simulink model "chairforceoneMV"  (R2024a)
settings: Solver=VariableStepAuto  StartTime=0.0  StopTime=1000.0  RelTol=1e-3
settings Model: Creator=sprinkle  LastModifiedBy=suryachand
settings OptimizationCC: ReuseModelBlockBuffer=off
settings RTWCC: GPUComputeCapability=3.5

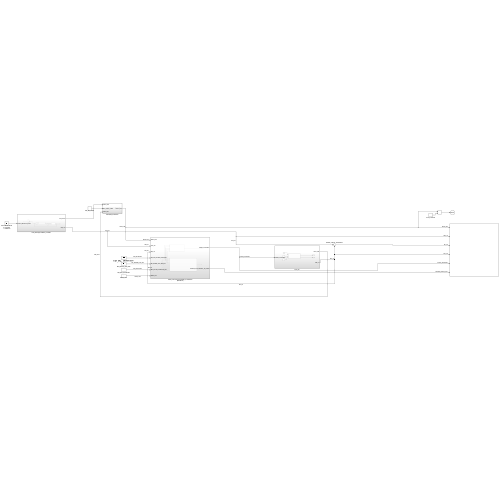
[thumbnail: Simulink's stored preview of the top-level diagram]
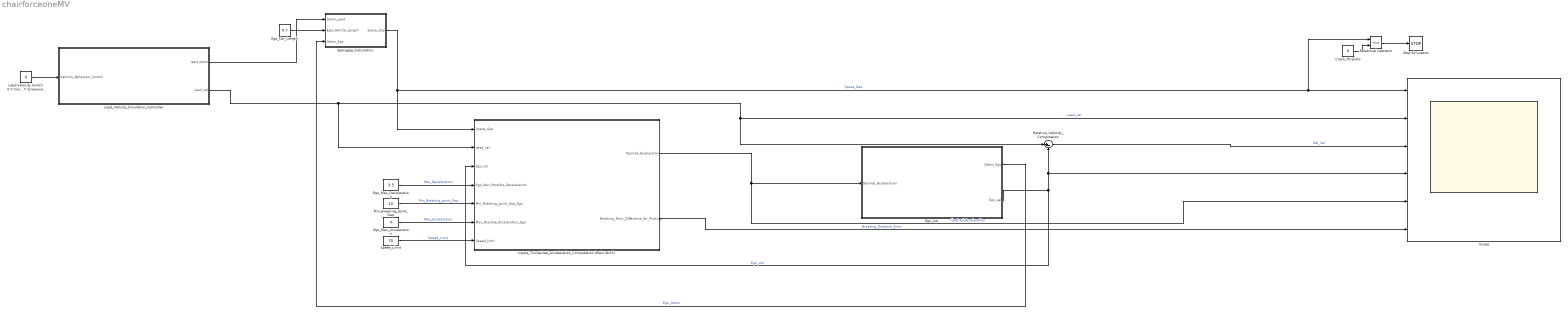
== system chairforceoneMV ==
  Crash_Thrshold : Constant  Value=0
  Ego_Car : Subsystem
  Ego_Car_Length : Constant  Value=4.7
  Ego_Max_Acceleration : Constant  Value=4
  "Ego_Max_Deceleration " : Constant  Value=3.5
  Inputs_To-Desired_Acceleration_Computation (Main Work) : Subsystem
  "Lead Velocity Switch 0 = Constant 1 = Sinewave " : Constant  Value=0
  Lead_Vehicle_Simulation_Controller : Subsystem
  Min_Breaking_point_Gap : Constant  Value=10
  Relational Operator : RelationalOperator  Operator=<=  OutDataTypeStr=boolean  RndMeth=Simplest  InputSameDT=off
  Relative_Velocity_Computation : Sum  Inputs=|+-
  Scope : Scope  NumInputPorts=6
  Spacegap_Calculation : Subsystem
  Speed_Limit : Constant  Value=70
  Stop Simulation : Stop
  wires:
  Relative_Velocity_Computation/1 -> Scope/3  "Rel_Vel"
  Lead_Vehicle_Simulation_Controller/2(lead_vel) -> Relative_Velocity_Computation/1, Scope/2, Inputs_To-Desired_Acceleration_Computation (Main Work)/2(Lead_vel)  "Lead_vel"
  "Lead Velocity Switch 0 = Constant 1 = Sinewave "/1 -> Lead_Vehicle_Simulation_Controller/1(Velocity_Behaviour_Switch)
  Spacegap_Calculation/1(Space_Gap) -> Inputs_To-Desired_Acceleration_Computation (Main Work)/1(Space_Gap), Relational Operator/1, Scope/1  "Space_Gap"
  Lead_Vehicle_Simulation_Controller/1(lead_odom) -> Spacegap_Calculation/1(Odom_Lead)
  Ego_Car_Length/1 -> Spacegap_Calculation/2(Ego_Vehicle_Length)
  Inputs_To-Desired_Acceleration_Computation (Main Work)/1(Desired_Acceleration) -> Scope/5, Ego_Car/1(Desired_Acceleration)  "Desired_Acceleration"
  "Ego_Max_Deceleration "/1 -> Inputs_To-Desired_Acceleration_Computation (Main Work)/4(Ego_Max_Possible_Deceleration)  "Max_Deceleration"
  Min_Breaking_point_Gap/1 -> Inputs_To-Desired_Acceleration_Computation (Main Work)/5(Min_Breaking_point_Gap_Ego)  "Min_Breaking_point_Gap"
  Ego_Car/2(Ego_vel) -> Relative_Velocity_Computation/2, Scope/4, Inputs_To-Desired_Acceleration_Computation (Main Work)/3(Ego_vel)  "Ego_Vel"
  Ego_Car/1(Odom_Ego) -> Spacegap_Calculation/3(Odom_Ego)  "Ego_Odom"
  Ego_Max_Acceleration/1 -> Inputs_To-Desired_Acceleration_Computation (Main Work)/6(Max_Possible_Acceleration_Ego)  "Max_Acceleration"
  Inputs_To-Desired_Acceleration_Computation (Main Work)/2(Breaking_Point_Difference_for_Plotting) -> Scope/6  "Breaking_Distance_Error"
  Speed_Limit/1 -> Inputs_To-Desired_Acceleration_Computation (Main Work)/7(Speed_limit)  "Speed_Limit"
  Relational Operator/1 -> Stop Simulation/1
  Crash_Thrshold/1 -> Relational Operator/2

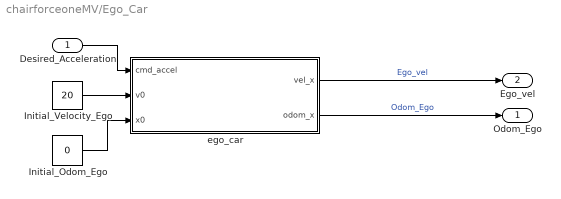
== system chairforceoneMV/Ego_Car ==
  Desired_Acceleration : Inport
  Initial_Odom_Ego : Constant  Value=0
  Initial_Velocity_Ego : Constant  Value=20
  ego_car : Subsystem
  Odom_Ego : Outport
  Ego_vel : Outport  Port=2
  wires:
  ego_car/2(odom_x) -> Odom_Ego/1  "Odom_Ego"
  ego_car/1(vel_x) -> Ego_vel/1  "Ego_vel"
  Initial_Odom_Ego/1 -> ego_car/3(x0)
  Desired_Acceleration/1 -> ego_car/1(cmd_accel)
  Initial_Velocity_Ego/1 -> ego_car/2(v0)

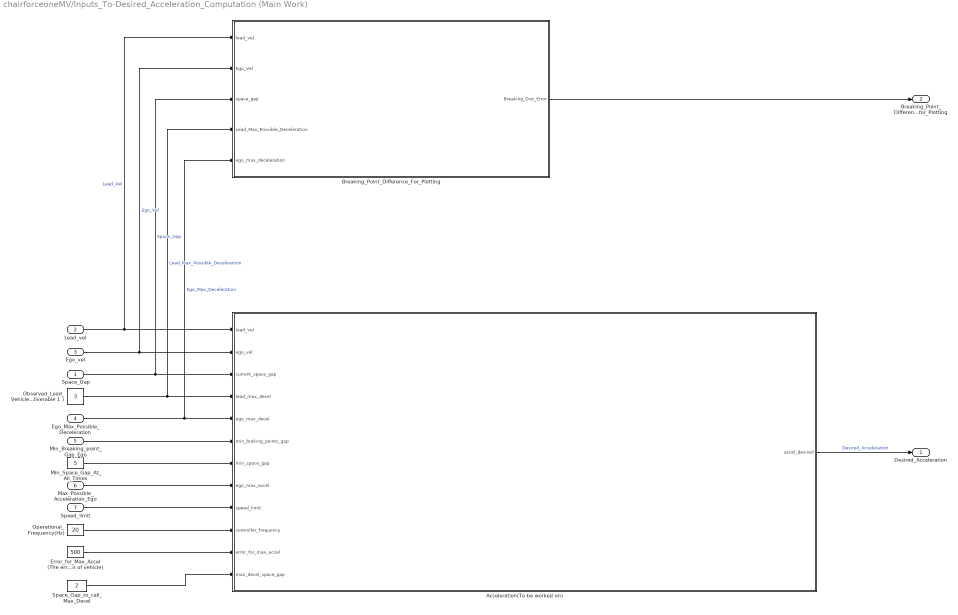
== system chairforceoneMV/Inputs_To-Desired_Acceleration_Computation (Main Work) ==
  Space_Gap : Inport
  Lead_vel : Inport  Port=2
  Ego_vel : Inport  Port=3
  Ego_Max_Possible_Deceleration : Inport  Port=4
  Min_Breaking_point_Gap_Ego : Inport  Port=5
  Max_Possible_Acceleration_Ego : Inport  Port=6
  Speed_limit : Inport  Port=7
  Acceleration(To be worked on) : MATLAB Function  TreatAsAtomicUnit=on
  Breaking_Point_Difference_For_Plotting : Subsystem
  Error_for_Max_Accel (The error distance in breaking points which is threshold for using max acceleration of vehicle) : Constant  Value=500
  Min_Space_Gap_At_All_Times : Constant  Value=5
  Observed_Lead_Vehicle_Max_Deceleration (For now keeping one fixed value to all vehicles for scope of deliverable 1 ) : Constant  Value=3
  Operational_Frequency(Hz) : Constant  Value=20
  Space_Gap_to_call_Max_Decel : Constant  Value=2
  Desired_Acceleration : Outport
  Breaking_Point_Difference_for_Plotting : Outport  Port=2
  wires:
  Acceleration(To be worked on)/1(accel_desired) -> Desired_Acceleration/1  "Desired_Acceleration"
  Min_Breaking_point_Gap_Ego/1 -> Acceleration(To be worked on)/6(min_braking_points_gap)
  Max_Possible_Acceleration_Ego/1 -> Acceleration(To be worked on)/8(ego_max_accel)
  Speed_limit/1 -> Acceleration(To be worked on)/9(speed_limit)
  Min_Space_Gap_At_All_Times/1 -> Acceleration(To be worked on)/7(min_space_gap)
  Operational_Frequency(Hz)/1 -> Acceleration(To be worked on)/10(controller_frequency)
  Error_for_Max_Accel (The error distance in breaking points which is threshold for using max acceleration of vehicle)/1 -> Acceleration(To be worked on)/11(error_for_max_accel)
  Space_Gap_to_call_Max_Decel/1 -> Acceleration(To be worked on)/12(max_decel_space_gap)
  Space_Gap/1 -> Acceleration(To be worked on)/3(current_space_gap), Breaking_Point_Difference_For_Plotting/3(space_gap)  "Space_Gap"
  Ego_Max_Possible_Deceleration/1 -> Acceleration(To be worked on)/5(ego_max_decel), Breaking_Point_Difference_For_Plotting/5(ego_max_deceleration)  "Ego_Max_Deceleration"
  Observed_Lead_Vehicle_Max_Deceleration (For now keeping one fixed value to all vehicles for scope of deliverable 1 )/1 -> Acceleration(To be worked on)/4(lead_max_decel), Breaking_Point_Difference_For_Plotting/4(Lead_Max_Possible_Deceleration)  "Lead_Max_Possible_Deceleration"
  Ego_vel/1 -> Acceleration(To be worked on)/2(ego_vel), Breaking_Point_Difference_For_Plotting/2(Ego_Vel)  "Ego_Vel"
  Lead_vel/1 -> Acceleration(To be worked on)/1(lead_vel), Breaking_Point_Difference_For_Plotting/1(lead_vel)  "Lead_Vel"
  Breaking_Point_Difference_For_Plotting/1(Breaking_Dist_Error) -> Breaking_Point_Difference_for_Plotting/1

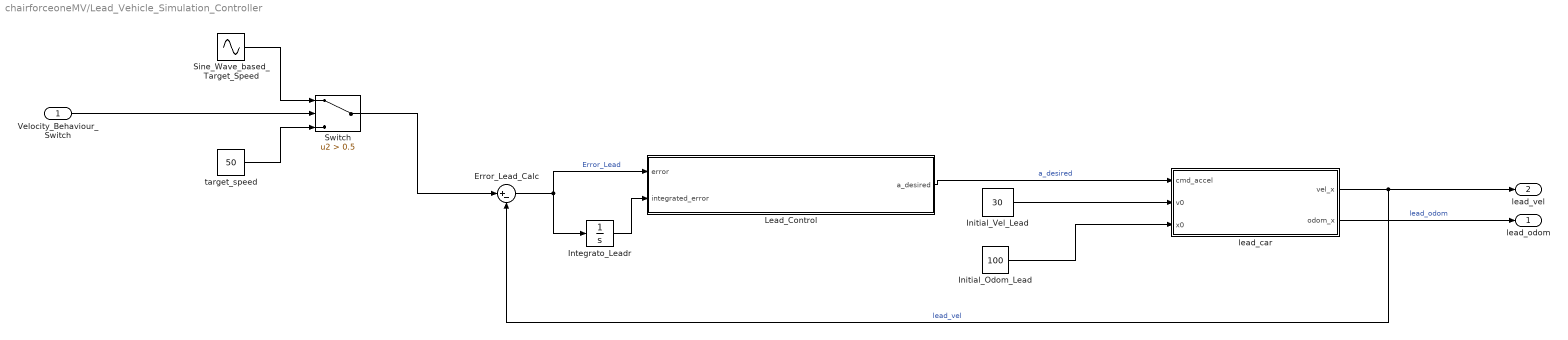
== system chairforceoneMV/Lead_Vehicle_Simulation_Controller ==
  Velocity_Behaviour_Switch : Inport
  Error_Lead_Calc : Sum  Inputs=|+-
  Initial_Odom_Lead : Constant  Value=100
  Initial_Vel_Lead : Constant  Value=30
  Integrato_Leadr : Integrator
  Lead_Control : MATLAB Function  TreatAsAtomicUnit=on
  Sine_Wave_based_Target_Speed : Sin  Amplitude=5  Bias=50  SampleTime=0
  Switch : Switch  Criteria=u2 > Threshold  Threshold=0.5  SaturateOnIntegerOverflow=off  InputSameDT=off
  lead_car : Subsystem
  target_speed : Constant  Value=50
  lead_odom : Outport
  lead_vel : Outport  Port=2
  wires:
  Velocity_Behaviour_Switch/1 -> Switch/2
  lead_car/1(vel_x) -> Error_Lead_Calc/2, lead_vel/1  "lead_vel"
  lead_car/2(odom_x) -> lead_odom/1  "lead_odom"
  Switch/1 -> Error_Lead_Calc/1
  Integrato_Leadr/1 -> Lead_Control/2(integrated_error)
  Initial_Vel_Lead/1 -> lead_car/2(v0)
  target_speed/1 -> Switch/3
  Error_Lead_Calc/1 -> Integrato_Leadr/1, Lead_Control/1(error)  "Error_Lead"
  Initial_Odom_Lead/1 -> lead_car/3(x0)
  Lead_Control/1(a_desired) -> lead_car/1(cmd_accel)  "a_desired"
  Sine_Wave_based_Target_Speed/1 -> Switch/1

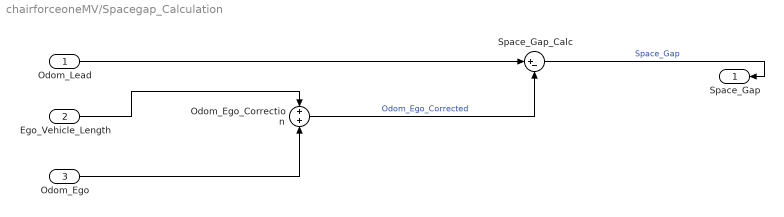
== system chairforceoneMV/Spacegap_Calculation ==
  Odom_Lead : Inport
  Ego_Vehicle_Length : Inport  Port=2
  Odom_Ego : Inport  Port=3
  Odom_Ego_Correction : Sum
  Space_Gap_Calc : Sum  Inputs=|+-
  Space_Gap : Outport
  wires:
  Odom_Ego/1 -> Odom_Ego_Correction/2
  Odom_Lead/1 -> Space_Gap_Calc/1
  Ego_Vehicle_Length/1 -> Odom_Ego_Correction/1
  Space_Gap_Calc/1 -> Space_Gap/1  "Space_Gap"
  Odom_Ego_Correction/1 -> Space_Gap_Calc/2  "Odom_Ego_Corrected"

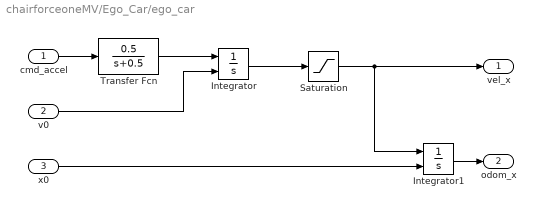
== system chairforceoneMV/Ego_Car/ego_car ==
  cmd_accel : Inport
  v0 : Inport  Port=2
  x0 : Inport  Port=3
  Integrator : Integrator  InitialConditionSource=external
  Integrator1 : Integrator  InitialConditionSource=external
  Saturation : Saturate  UpperLimit=80  LowerLimit=0
  Transfer Fcn : TransferFcn  Numerator=[0.5]  Denominator=[1 0.5]
  vel_x : Outport
  odom_x : Outport  Port=2
  wires:
  v0/1 -> Integrator/2
  cmd_accel/1 -> Transfer Fcn/1
  Transfer Fcn/1 -> Integrator/1
  Integrator1/1 -> odom_x/1
  Integrator/1 -> Saturation/1
  x0/1 -> Integrator1/2
  Saturation/1 -> vel_x/1, Integrator1/1

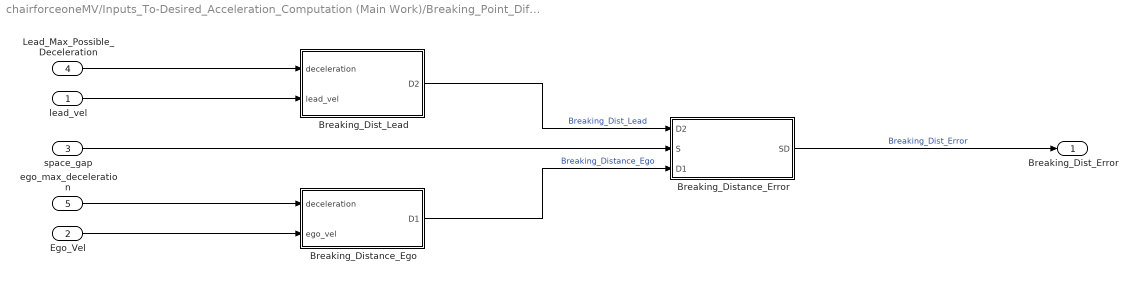
== system chairforceoneMV/Inputs_To-Desired_Acceleration_Computation (Main Work)/Breaking_Point_Difference_For_Plotting ==
  lead_vel : Inport
  Ego_Vel : Inport  Port=2
  space_gap : Inport  Port=3
  Lead_Max_Possible_Deceleration : Inport  Port=4
  ego_max_deceleration : Inport  Port=5
  Breaking_Dist_Lead : MATLAB Function  TreatAsAtomicUnit=on
  Breaking_Distance_Ego : MATLAB Function  TreatAsAtomicUnit=on
  Breaking_Distance_Error : MATLAB Function  TreatAsAtomicUnit=on
  Breaking_Dist_Error : Outport
  wires:
  Ego_Vel/1 -> Breaking_Distance_Ego/2(ego_vel)
  space_gap/1 -> Breaking_Distance_Error/2(S)
  lead_vel/1 -> Breaking_Dist_Lead/2(lead_vel)
  ego_max_deceleration/1 -> Breaking_Distance_Ego/1(deceleration)
  Breaking_Distance_Error/1(SD) -> Breaking_Dist_Error/1  "Breaking_Dist_Error"
  Breaking_Distance_Ego/1(D1) -> Breaking_Distance_Error/3(D1)  "Breaking_Distance_Ego"
  Lead_Max_Possible_Deceleration/1 -> Breaking_Dist_Lead/1(deceleration)
  Breaking_Dist_Lead/1(D2) -> Breaking_Distance_Error/1(D2)  "Breaking_Dist_Lead"

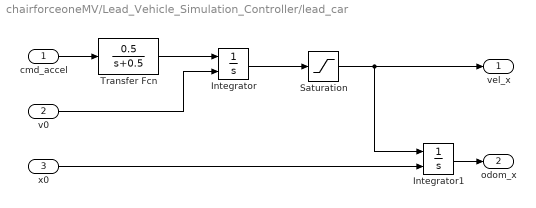
== system chairforceoneMV/Lead_Vehicle_Simulation_Controller/lead_car ==
  cmd_accel : Inport
  v0 : Inport  Port=2
  x0 : Inport  Port=3
  Integrator : Integrator  InitialConditionSource=external
  Integrator1 : Integrator  InitialConditionSource=external
  Saturation : Saturate  UpperLimit=80  LowerLimit=0
  Transfer Fcn : TransferFcn  Numerator=[0.5]  Denominator=[1 0.5]
  vel_x : Outport
  odom_x : Outport  Port=2
  wires:
  v0/1 -> Integrator/2
  cmd_accel/1 -> Transfer Fcn/1
  Transfer Fcn/1 -> Integrator/1
  Integrator1/1 -> odom_x/1
  Integrator/1 -> Saturation/1
  x0/1 -> Integrator1/2
  Saturation/1 -> vel_x/1, Integrator1/1

== matlab function chairforceoneMV/Inputs_To-Desired_Acceleration_Computation (Main Work)/Acceleration(To be worked on) ==
  data: accel_desired output; lead_vel input; ego_vel input; current_space_gap input; lead_max_decel input; ego_max_decel input; min_braking_points_gap input; min_space_gap input; ego_max_accel input; speed_limit input; controller_frequency input; error_for_max_accel input; max_decel_space_gap input
function accel_desired = accel_ctrl_(lead_vel, ego_vel, current_space_gap, ...
    lead_max_decel, ego_max_decel, min_braking_points_gap, min_space_gap, ...
    ego_max_accel, speed_limit, controller_frequency, error_for_max_accel, max_decel_space_gap)
    % ACCEL_CTRL_ Calculates the desired acceleration for the ego vehicle to maintain
    % a safe following distance behind a lead vehicle while considering vehicle capabilities
    % and safety constraints.
    %
    % Parameters:
    %   lead_vel                - Velocity of the lead vehicle (m/s)
    %   ego_vel                 - Current velocity of the ego vehicle (m/s)
    %   current_space_gap       - Current distance between ego and lead vehicles (m)
    %   lead_max_decel          - Maximum deceleration capability of the lead vehicle (m/s²)
    %   ego_max_decel           - Maximum deceleration capability of the ego vehicle (m/s²)
    %   min_braking_points_gap  - Minimum desired gap based on braking points (m)
    %   min_space_gap           - Absolute minimum safe space gap (m)
    %   ego_max_accel           - Maximum acceleration capability of the ego vehicle (m/s²)
    %   speed_limit             - Speed limit of the road (m/s) [Not used in current implementation]
    %   controller_frequency    - Frequency at which the controller operates (Hz)
    %   error_for_max_accel     - Error threshold at which maximum acceleration is applied (m)
    %   max_decel_space_gap     - Additional space gap for maximum deceleration (m)
    %
    % Returns:
    %   accel_desired - The desired acceleration command for the ego vehicle (m/s²)
    
    % Constants
    f = 0.55; % Coefficient of friction between tires and road
    g = 9.8;  % Acceleration due to gravity (m/s²)

    % Time step calculation based on controller frequency
    dt = 1 / controller_frequency;

    % Step 1: Initialize Working Variables
    % -------------------------------------
    % These variables may be adjusted based on the relative deceleration capabilities
    % of the ego and lead vehicles.
    working_decel_ego = ego_max_decel;   % Working maximum deceleration of ego vehicle
    working_decel_lead = lead_max_decel; % Working maximum deceleration of lead vehicle
    working_min_gap = min_braking_points_gap; % Minimum braking point gap

    % Conditional Adjustment Based on Maximum Decelerations
    if ego_max_decel > lead_max_decel
        % If ego vehicle can decelerate faster than lead vehicle,
        % limit ego's deceleration to lead's maximum deceleration to maintain safety.
        working_decel_ego = lead_max_decel;

        % Adjust the working minimum gap to ensure safety
        working_min_gap = min(min_space_gap, min_braking_points_gap);
    end

    % Step 2: Calculate Stopping Distances
    % -------------------------------------
    % Calculate the stopping distances for both ego and lead vehicles.
    % The stopping distance accounts for both the distance required to stop and
    % the distance covered due to friction.
    D1 = (ego_vel^2 / (2 * working_decel_ego)) + ((ego_vel^2 / (2 * g)) * f);
    D2 = (lead_vel^2 / (2 * working_decel_lead)) + ((lead_vel^2 / (2 * g)) * f);

    % Step 3: Compute the Stopping Distance Error
    % -------------------------------------------
    % Determine how much the current stopping distance deviates from the desired minimum gap.
    stop_dist = (D2 + current_space_gap) - D1;
    error = stop_dist - working_min_gap;

    % Step 4: Map Error to Desired Acceleration Using Different Gamma Values
    % ------------------------------------------------------------------------
    % Depending on whether the error indicates a need to accelerate or decelerate,
    % apply different responsiveness levels using gamma values.
    % gamma_neg controls responsiveness during deceleration.
    % gamma_pos controls responsiveness during acceleration.
    gamma_neg = 1; % For deceleration (negative errors)
    gamma_pos = 2; % For acceleration (positive errors)

    % Define Thresholds for Applying Maximum Acceleration or Deceleration
    threshold_decel_error = -(working_min_gap - max_decel_space_gap); % Negative threshold
    threshold_accel_error = error_for_max_accel; % Positive threshold

    if error >= threshold_accel_error
        % Case 1: Error exceeds the positive threshold
        % Apply maximum acceleration.
        accel_desired = ego_max_accel;
    elseif error >= 0
        % Case 2: Error is positive but below the threshold
        % Apply a non-linear (quadratic) mapping to determine desired acceleration.
        accel_desired = ego_max_accel * (error / threshold_accel_error)^gamma_pos;
    elseif error <= threshold_decel_error
        % Case 3: Error exceeds the negative threshold
        % Apply maximum deceleration.
        accel_desired = -ego_max_decel;
    else
        % Case 4: Error is negative but above the threshold
        % Apply a non-linear (linear in this case) mapping to determine desired deceleration.
        % The fraction (error / threshold_decel_error) is positive.
        accel_desired = -ego_max_decel * (error / threshold_decel_error)^gamma_neg;
    end

    % Step 5: One-Step Lookahead
    % ---------------------------
    % Predict the future positions of both ego and lead vehicles after one time step (dt)
    % to ensure that the desired acceleration maintains a safe following distance.
    
    % Predict Future Position of Ego Vehicle
    % Using the kinematic equation: s = ut + 0.5 * a * t²
    ego_future_pos = ego_vel * dt + 0.5 * accel_desired * dt^2; % Assuming current position is 0

    % Predict Future Position of Lead Vehicle
    % Assuming the lead vehicle maintains constant velocity.
    lead_future_pos = current_space_gap + lead_vel * dt;

    % Compute Future Space Gap Between Lead and Ego Vehicles
    future_space_gap = lead_future_pos - ego_future_pos;

    % Adjust Desired Acceleration if Future Space Gap is Less Than Minimum Safe Gap
    if future_space_gap < min_space_gap
        % Calculate the required acceleration to maintain the minimum space gap.
        delta_s = (current_space_gap + lead_vel * dt) - (ego_vel * dt + min_space_gap);
        accel_required = (2 * (delta_s - ego_vel * dt)) / dt^2;

        % Adjust accel_desired to prevent collision by choosing the smaller acceleration.
        accel_desired = min(accel_required, accel_desired);

        % Ensure accel_desired remains within the vehicle's acceleration limits.
        accel_desired = min(accel_desired, ego_max_accel);
        accel_desired = max(accel_desired, -ego_max_decel);
    end

    % Step 6: Final Clipping of Desired Acceleration
    % -----------------------------------------------
    % Ensure that the calculated desired acceleration does not exceed the vehicle's
    % physical capabilities by clipping it within the allowable range.
    accel_desired = min(accel_desired, ego_max_accel);    % Limit to maximum acceleration
    accel_desired = max(accel_desired, -ego_max_decel);   % Limit to maximum deceleration
end

== matlab function chairforceoneMV/Lead_Vehicle_Simulation_Controller/Lead_Control ==
  data: error input; a_desired output; integrated_error input
function a_desired = controller(error,integrated_error)

a_desired = 0.3*error + 0.01*integrated_error;

== matlab function chairforceoneMV/Inputs_To-Desired_Acceleration_Computation (Main Work)/Breaking_Point_Difference_For_Plotting/Breaking_Distance_Error ==
  data: D2 input; SD output; S input; D1 input
function SD = stop_dist_diff(D2, S, D1)

SD = (D2+S)-D1;

== matlab function chairforceoneMV/Inputs_To-Desired_Acceleration_Computation (Main Work)/Breaking_Point_Difference_For_Plotting/Breaking_Distance_Ego ==
  data: deceleration input; D1 output; ego_vel input
function D1 = D1(deceleration, ego_vel)
    f=0.55; % coeff. friction
    g=9.8;
    D1 = (ego_vel^2 / (2*deceleration))+((ego_vel^2/(2*g))*f);

== matlab function chairforceoneMV/Inputs_To-Desired_Acceleration_Computation (Main Work)/Breaking_Point_Difference_For_Plotting/Breaking_Dist_Lead ==
  data: deceleration input; lead_vel input; D2 output
function D2 = D2(deceleration, lead_vel)
    f=0.55; % coeff. friction
    g=9.8;
    D2 = (lead_vel^2 / (2*deceleration))+((lead_vel^2/(2*g))*f);
